simulink model "simModel"  (R2019a)
settings: Solver=ode45  StartTime=0.0  StopTime=inf  FixedStep=uav.sampleTime  RelTol=1e-3  EnableMultiTasking=on
InitFcn:
  | plantConfigSet = sim_plant_configset;
libraries: aerolibanimutils x1, mbdriLib x1
settings Model: ParamWorkspaceSource=ReferencedWorkspace  Creator=mlizarra  LastModifiedBy=tyson
settings SolverCC: PositivePriorityOrder=on  AutoInsertRateTranBlk=on  DecoupledContinuousIntegration=on
settings DataIOCC: SaveOutput=off  DSMLogging=off
settings OptimizationCC: DefaultParameterBehavior=Inlined  UseDivisionForNetSlopeComputation=UseDivisionForReciprocalsOfIntegersOnly  DefaultUnderspecifiedDataType=single  InlineInvariantSignals=on  PassReuseOutputArgsAs=Individual arguments  StateBitsets=on  DataBitsets=on  ZeroExternalMemoryAtStartup=off  ZeroInternalMemoryAtStartup=off  InitFltsAndDblsToZero=on  LifeSpan=1  MaxStackSize=64
settings DebuggingCC: AlgebraicLoopMsg=error  ParameterPrecisionLossMsg=none  SFUnexpectedBacktrackingDiag=warning  SFNoUnconditionalDefaultTransitionDiag=warning  SFExecutionAtInitializationDiag=none  ArithmeticOperatorsInVariantConditions=warning
settings HardwareCC: ProdBitPerPointer=32  ProdBitPerSizeT=32  ProdBitPerPtrDiffT=32  ProdLargestAtomicInteger=Long  ProdLargestAtomicFloat=Double  ProdWordSize=32  ProdHWDeviceType=ARM Compatible->ARM Cortex
settings SFSimCC: SimUseLocalCustomCode=off  MATLABDynamicMemAlloc=off
settings RTWCC: SystemTargetFile=ert.tlc  HardwareBoard=Raspberry Pi  TLCOptions="-aInlineSetEventsForThisBaseRateFcn=TLC_FALSE -aSuppressMultiTaskScheduler=TLC_FALSE  -aRateBasedStepFcn=0"  TemplateMakefile=ert_default_tmf  GenerateReport=on  RTWUseLocalCustomCode=off  Toolchain=GNU GCC Raspberry Pi  IncludeHyperlinkInReport=on  LaunchReport=on  GenerateTraceInfo=on  GenerateTraceReport=on  GenerateTraceReportSl=on  GenerateTraceReportSf=on  GenerateTraceReportEml=on
settings CodeAppCC: ForceParamTrailComments=on  IgnoreCustomStorageClasses=off  OperatorAnnotations=on  SimulinkDataObjDesc=on  SFDataObjDesc=on  MATLABFcnDesc=on  InsertBlockDesc=on  StateflowObjectComments=on  MATLABSourceComments=on
settings ERTTargetCC: TargetLangStandard=C99 (ISO)  MultiwordLength=2048  SupportVariableSizeSignals=on
settings ConfigComp: CovMetricSettings=dw  CovHtmlReporting=on  CovSaveCumulativeToWorkspaceVar=on  CovSaveSingleToWorkspaceVar=on  CovExternalEMLEnable=off
settings SimscapeCC: SimscapeNormalizeSystem=off

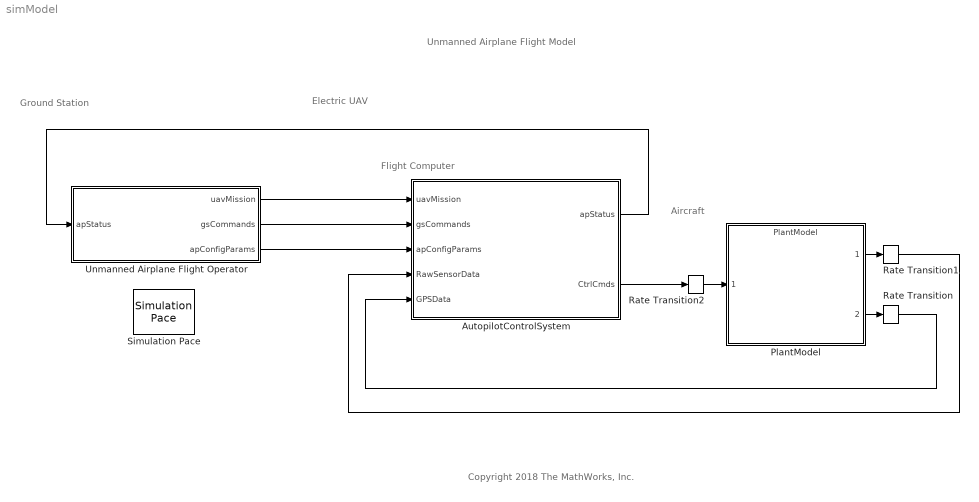
== system simModel ==
  note: Electric UAV
  note: Aircraft
  note: Flight Computer
  note: Copyright 2018 The MathWorks, Inc.
  note: Unmanned Airplane Flight Model
  note: Ground Station
  AutopilotControlSystem : Subsystem  Variant=on  VariantControl=Variant1
  PlantModel : ModelReference  ModelNameDialog=PlantModel  SimulationMode=Normal  ModelReferenceVersion=1.373
  Rate Transition : RateTransition  OutPortSampleTime=ap.apSampleTime
  Rate Transition1 : RateTransition  OutPortSampleTime=ap.apSampleTime
  Rate Transition2 : RateTransition
  Simulation Pace : aerolibanimutils/Simulation Pace  SimulationPace=1  SleepMode=MATLAB Thread  OutputPaceError=off  SampleTime=0.01
  "Unmanned Airplane Flight Operator " : Subsystem
  wires:
  PlantModel/1 -> Rate Transition1/1
  PlantModel/2 -> Rate Transition/1
  "Unmanned Airplane Flight Operator "/1(uavMission) -> AutopilotControlSystem/1("uavMission ")
  "Unmanned Airplane Flight Operator "/2(gsCommands) -> AutopilotControlSystem/2("gsCommands ")
  "Unmanned Airplane Flight Operator "/3(apConfigParams) -> AutopilotControlSystem/3("apConfigParams ")
  Rate Transition1/1 -> AutopilotControlSystem/4("RawSensorData ")
  Rate Transition/1 -> AutopilotControlSystem/5("GPSData ")
  AutopilotControlSystem/1(" apStatus") -> "Unmanned Airplane Flight Operator "/1(apStatus)
  AutopilotControlSystem/2(" CtrlCmds") -> Rate Transition2/1
  Rate Transition2/1 -> PlantModel/1

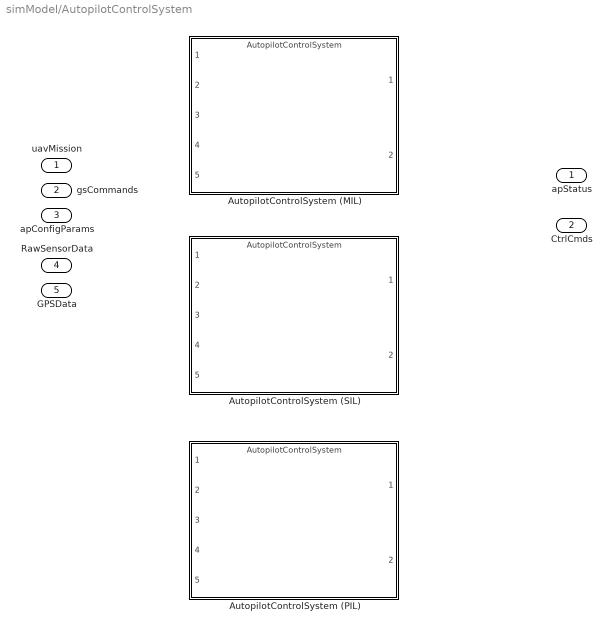
== system simModel/AutopilotControlSystem ==
  "uavMission " : Inport
  "gsCommands " : Inport  Port=2
  "apConfigParams " : Inport  Port=3
  "RawSensorData " : Inport  Port=4
  "GPSData " : Inport  Port=5
  AutopilotControlSystem (MIL) : ModelReference  ModelNameDialog=AutopilotControlSystem  SimulationMode=Normal  CodeInterface=Top model  VariantControl=MIL  ModelReferenceVersion=1.363
  AutopilotControlSystem (PIL) : ModelReference  ModelNameDialog=AutopilotControlSystem  SimulationMode=Processor-in-the-loop (PIL)  CodeInterface=Top model  VariantControl=PIL  ModelReferenceVersion=1.363
  AutopilotControlSystem (SIL) : ModelReference  ModelNameDialog=AutopilotControlSystem  SimulationMode=Software-in-the-loop (SIL)  CodeInterface=Top model  VariantControl=SIL  ModelReferenceVersion=1.363
  " apStatus" : Outport
  " CtrlCmds" : Outport  Port=2

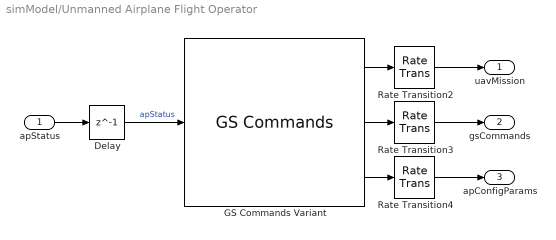
== system simModel/Unmanned Airplane Flight Operator  ==
  apStatus : Inport  OutDataTypeStr=Bus: apStatusBus
  Delay : Delay  DelayLength=1
  GS Commands Variant : mbdriLib/Utilities/GS Commands   SystemSampleTime=-1
      settings: SourceProductName=Robotics System Toolbox  SourceProductBaseCode=RO
  Rate Transition2 : RateTransition  OutPortSampleTime=ap.apSampleTime
  Rate Transition3 : RateTransition  OutPortSampleTime=ap.apSampleTime
  Rate Transition4 : RateTransition  OutPortSampleTime=ap.apSampleTime
  uavMission : Outport  OutDataTypeStr=Bus: waypoint
  gsCommands : Outport  Port=2  OutDataTypeStr=Bus: gsCommandsBus
  apConfigParams : Outport  Port=3  OutDataTypeStr=Bus: apConfigParamsBus
  wires:
  Rate Transition2/1 -> uavMission/1
  GS Commands Variant/3 -> Rate Transition4/1
  apStatus/1 -> Delay/1
  GS Commands Variant/2 -> Rate Transition3/1
  Delay/1 -> GS Commands Variant/1  "apStatus"
  GS Commands Variant/1 -> Rate Transition2/1
  Rate Transition4/1 -> apConfigParams/1
  Rate Transition3/1 -> gsCommands/1
